simulink model "main_raspi"  (R2017a)
settings: Solver=VariableStepAuto  StartTime=0.0  StopTime=10  RelTol=1e-3
undefined symbols (not defined in the file or in its folder): sigbuilder_block
settings Model: Creator=Vincent  LastModifiedBy=Vincent

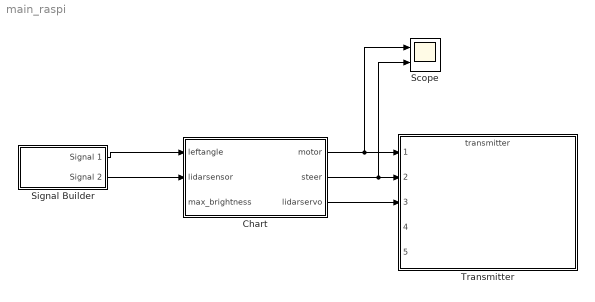
== system main_raspi ==
  Chart : Stateflow chart  TreatAsAtomicUnit=on
  Scope : Scope  NumInputPorts=2
  Signal Builder : Subsystem  Tag=STV Subsys  LoadFcn=sigbuilder_block('load');  StartFcn=sigbuilder_block('start');  StopFcn=sigbuilder_block('stop');  ClipboardFcn=sigbuilder_block('clipboard');  mask(Sigbuilder block){tuvar=[0:10]}
      mask help: Simulink:masks:SigbuilderBlock_MD
      mask init:
      | if ~strcmp(get_param(bdroot(gcbh),'SimulationStatus'),'stopped') tuvar = sigbuilder_block('maskInit'); end
      settings: CopyFcn=sigbuilder_block('copy');  DeleteFcn=sigbuilder_block('delete');  ModelCloseFcn=sigbuilder_block('modelClose');  PreSaveFcn=sigbuilder_block('preSave');  PauseFcn=sigbuilder_block('pause');  ContinueFcn=sigbuilder_block('continue');  NameChangeFcn=sigbuilder_block('namechange');  OpenFcn=sigbuilder_block('open',[437.6 199.2 550.4 400 ]);  CloseFcn=sigbuilder_block('close');
      mask Display: plot(0, 0, 100, 100,[2, 2, 32, 32, 2], [68, 8, 8, 68, 68],[32, 2], [38, 38], [32, 19, 2],[53, 60, 44], [32, 17, 17, 2],[16, 16, 31, 31]);txt = getActiveGroup(gcbh);text(2, 100, txt,'verticalAlignment', 'top');
  Transmitter : ModelReference  ModelNameDialog=transmitter.slx  SimulationMode=Normal  ModelReferenceVersion=1.10
  wires:
  Chart/1(motor) -> Scope/1, Transmitter/1
  Chart/2(steer) -> Scope/2, Transmitter/2
  Chart/3(lidarservo) -> Transmitter/3
  Signal Builder/1(Signal 1) -> Chart/1(leftangle)
  Signal Builder/2(Signal 2) -> Chart/2(lidarsensor)

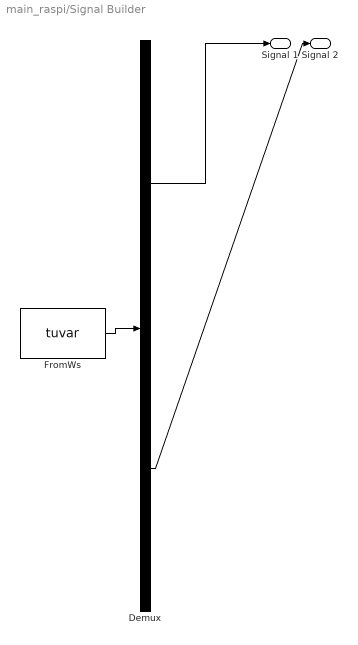
== system main_raspi/Signal Builder ==
  Demux : Demux  Tag=STV Demux  Outputs=2
  FromWs : FromWorkspace  Tag=STV FromWs  VariableName=tuvar  SampleTime=0
      SigBuilderData=|
      | common.afterFinalStr = 'Extrapolate'
      | common.sampleTime = 0
      | dataSet.timeRange = [0 10]
      | dataSet.name = 'Group 1'
      | sbobj.Groups.Name = 'Group 1'
      | sbobj.Groups.Signals(1).Name = 'Signal 1'
      | sbobj.Groups.Signals(1).XData = [0 3 4.45 5.05 6 7 9 10]
      | sbobj.Groups.Signals(1).YData = [45 45 48 -4 -3 43 45 45]
      | sbobj.Groups.Signals(2).Name = 'Signal 2'
      | sbobj.Groups.Signals(2).XData = [0 4 5 6 6 10]
      | sbobj.Groups.Signals(2).YData = [300 295 25 1 0 300]
  Signal 1 : Outport  Tag=STV Outport
  Signal 2 : Outport  Tag=STV Outport  Port=2
  wires:
  Demux/1 -> Signal 1/1
  FromWs/1 -> Demux/1
  Demux/2 -> Signal 2/1

== stateflow chart main_raspi/Chart ==
  state init
    entry:
    commonangle = leftangle;
    motor = 20;
    steer = 0;
    lidarservo = 0;
  state init_tunnel
    entry:
    lidarservo = -90;
    steer = 0;
    motor = 25;
  state forward
    entry:
    saveangle = leftangle;
    motor = motor + 2;
    steer = 0;
    lidarservo = 0;
  state evade_obstacle
    entry:
    saveangle = leftangle;
    motor = motor + 2;
    steer = 50;
  state forward_tunnel
    entry:
    steer = 0;
    motor = 25;
  state steady
    entry:
    saveangle = leftangle;
    motor = motor - abs(saveangle-commonangle)/4;
    steer = steer - (saveangle-commonangle)/4;
    lidarservo = lidarservo + (saveangle-commonangle)/4;
  state wait_to_return
    entry:
    lidarservo = -90;
    steer = 0;
  state turnright_tunnel
    entry:
    steer = 15;
    motor = motor - 1;
  state return_to_lane
    entry:
    saveangle = leftangle;
    motor = motor + 2;
    steer = -50;
  (default) -> init
  init -> forward
  forward -> forward [order 4]
  forward -> init_tunnel [order 2] : [max_brightness < 50]
  init_tunnel -> forward_tunnel
  forward -> evade_obstacle [order 1] : [lidarsensor < 25]
  return_to_lane -> forward : [saveangle >= 20 && saveangle <=70]
  steady -> forward [order 2] : [abs(saveangle - commonangle) < 2]
  forward -> steady [order 3] : [abs(saveangle - commonangle) >= 2]
  steady -> evade_obstacle [order 1] : [lidarsensor < 25]
  evade_obstacle -> wait_to_return : [saveangle >= 20 && saveangle <=70]
  forward_tunnel -> forward_tunnel [order 2]
  steady -> steady [order 3]
  wait_to_return -> return_to_lane : [lidarsensor >= 25]
  turnright_tunnel -> forward_tunnel [order 1] : [lidarsensor >= 8]
  forward_tunnel -> turnright_tunnel [order 1] : [lidarsensor < 8]
  turnright_tunnel -> turnright_tunnel [order 2]
  data: leftangle input size=1; lidarsensor input size=1; motor output size=1; steer output size=1; lidarservo output size=1; commonangle local; saveangle local; newsteer local; max_brightness input size=1
